simulink library "mbed_targets_stm_nucleo_f303"  (R2014a)
settings: Solver=ode45  StartTime=0.0  StopTime=10.0  RelTol=1e-3
libraries: mbed_lib x5
settings Model: Creator=oh  LastModifiedBy=oh

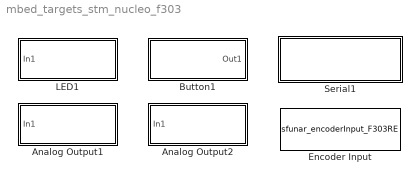
== system mbed_targets_stm_nucleo_f303 ==
  Analog Output1 : Subsystem  mask{Parameter1=0}
      mask Display:
      | offset=0.7;
      | plot([0+offset:0.025:0.25+offset],0.3*sin(2*pi*[0:0.1:1])+0.5)
      | port_label('input',1,['DAC1 (PA.4)']);
  Analog Output2 : Subsystem
      mask Display:
      | offset=0.7;
      | plot([0+offset:0.025:0.25+offset],0.3*sin(2*pi*[0:0.1:1])+0.5)
      | port_label('input',1,['DAC2 (PA.5)']);
  Button1 : Subsystem  mask{Parameter1=0}
      mask Display:
      | plot([0 0.15 0.15 0.35 0.35 0.5],[0.3 0.3 0.7 0.7 0.3 0.3])
      | port_label('output',1,['UsrBtn1']);
  Encoder Input : S-Function  FunctionName=sfunar_encoderInput_F303RE  Parameters=SampleTime, uint8(SParameter1), uint8(SParameter2), uint8(SParameter3), uint16(SParameter4)  EnableBusSupport=off  mask{SParameter1=TIM1, SParameter2=TI1, SParameter3=PullNone, SParameter4=65535, SampleTime=-1}
      mask prompts: SParameter1 "Timer number:"; SParameter2 "Encoder Mode:"; SParameter3 "Input Mode:"; SParameter4 "Resolution (Pulses/Rev):"; SampleTime "Sample time: (-1 for inherited)"
      mask TypeOptions SParameter1: TIM1 | TIM3 | TIM4 | TIM8
      mask TypeOptions SParameter2: TI1 | TI2 | TI1 and TI2
      mask TypeOptions SParameter3: PullNone | PullUp | PullDown
      mask DialogControl DescTextVar Prompt: Hardware Encoder für STM32F4xx
      mask Display:
      | port_label('input',1,'Reset');
      | disp(['Timer ' num2str(SParameter1)]);
      | port_label('output',1,'Angle');
      | port_label('output',2,'RAW');
  LED1 : Subsystem  mask{Parameter1=0}
      mask Display:
      | plot([0.5 0.65 0.65 0.85 0.85 1],[0.3 0.3 0.7 0.7 0.3 0.3])
      | port_label('input',1,['LED1']);
  Serial1 : Subsystem  mask{Parameter1=0}
      mask Display: disp(['Serial1(USB)\nTX:PA_2, RX:PA_3'])

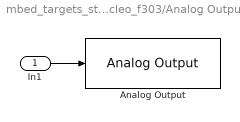
== system mbed_targets_stm_nucleo_f303/Analog Output1 ==
  In1 : Inport
  Analog Output : mbed_lib/GPIO/Analog Output  SParameter2=A  SParameter1=4  inputVariant=Double: 0 - 1.0f  SampleTime=-1
  wires:
  In1/1 -> Analog Output/1

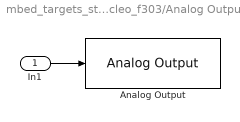
== system mbed_targets_stm_nucleo_f303/Analog Output2 ==
  In1 : Inport
  Analog Output : mbed_lib/GPIO/Analog Output  SParameter2=A  SParameter1=5  inputVariant=Double: 0 - 1.0f  SampleTime=-1
  wires:
  In1/1 -> Analog Output/1

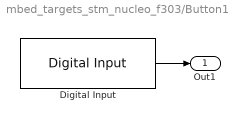
== system mbed_targets_stm_nucleo_f303/Button1 ==
  Digital Input : mbed_lib/GPIO/Digital Input  SParameter2=C  SParameter1=13  SParameter3=PullDefault  SampleTime=-1
  Out1 : Outport
  wires:
  Digital Input/1 -> Out1/1

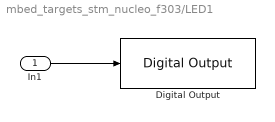
== system mbed_targets_stm_nucleo_f303/LED1 ==
  In1 : Inport
  Digital Output : mbed_lib/GPIO/Digital Output  SParameter2=A  SParameter1=5  SParameter3=PullDefault  SampleTime=-1
  wires:
  In1/1 -> Digital Output/1

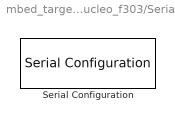
== system mbed_targets_stm_nucleo_f303/Serial1 ==
  Serial Configuration : mbed_lib/Serial/Serial Configuration  SerialPort=1  TXPort=A  TXPin=2  RXPort=A  RXPin=3  BaudRate=9600
